simulink model "simulink_qpsk_mrc"  (R2022b)
settings: Solver=VariableStepAuto  StartTime=0.0  StopTime=0  RelTol=1e-3
values from neighbouring files (symbols this model uses):
  n_sd = 1/sqrt(snrlin)    [sim_qpsk_mrc.m]    (also in task2.m = 1./sqrt(snr_lin(i)); task3.m = n(i))
settings Model: Creator=DSP-29  LastModifiedBy=DSP-29

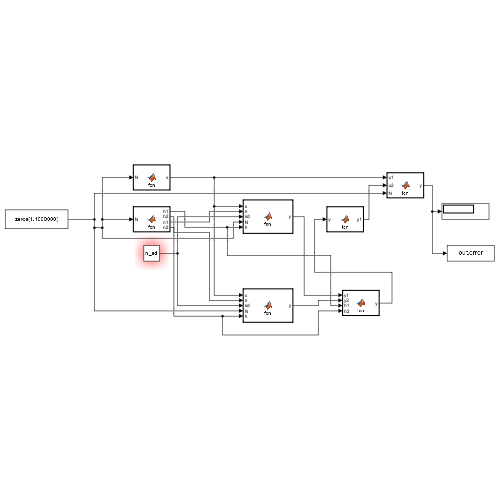
[thumbnail: Simulink's stored preview of the top-level diagram]
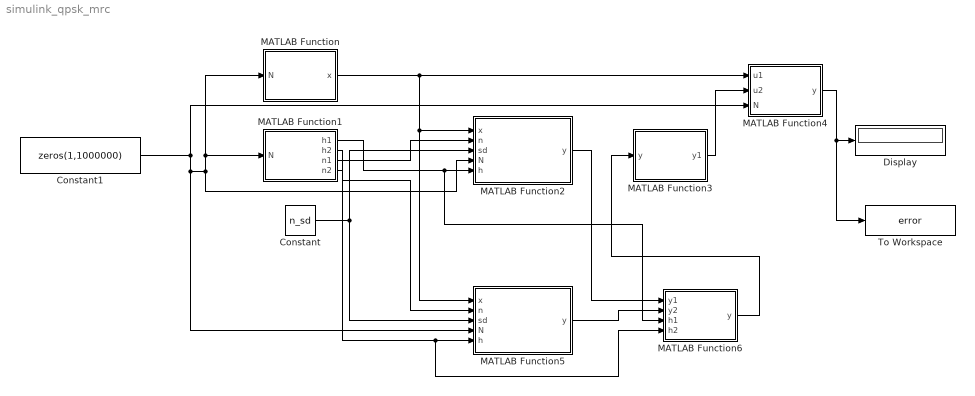
== system simulink_qpsk_mrc ==
  Constant : Constant  Value=n_sd
  Constant1 : Constant  Value=zeros(1,1000000)
  Display : Display
  MATLAB Function : MATLAB Function  TreatAsAtomicUnit=on
  MATLAB Function1 : MATLAB Function  TreatAsAtomicUnit=on
  MATLAB Function2 : MATLAB Function  TreatAsAtomicUnit=on
  MATLAB Function3 : MATLAB Function  TreatAsAtomicUnit=on
  MATLAB Function4 : MATLAB Function  TreatAsAtomicUnit=on
  MATLAB Function5 : MATLAB Function  TreatAsAtomicUnit=on
  MATLAB Function6 : MATLAB Function  TreatAsAtomicUnit=on
  To Workspace : ToWorkspace  VariableName=error  SampleTime=-1
      settings: Save2DSignal=2-D array (concatenate along first dimension)
  wires:
  MATLAB Function2/1(y) -> MATLAB Function6/1(y1)
  MATLAB Function1/1(h1) -> MATLAB Function6/3(h1), MATLAB Function2/5(h)
  MATLAB Function6/1(y) -> MATLAB Function3/1(y)
  Constant1/1 -> MATLAB Function5/4(N), MATLAB Function/1(N), MATLAB Function1/1(N), MATLAB Function2/4(N), MATLAB Function4/3(N)
  MATLAB Function4/1(y) -> To Workspace/1, Display/1
  MATLAB Function/1(x) -> MATLAB Function5/1(x), MATLAB Function2/1(x), MATLAB Function4/1(u1)
  Constant/1 -> MATLAB Function5/3(sd), MATLAB Function2/3(sd)
  MATLAB Function1/3(n1) -> MATLAB Function2/2(n)
  MATLAB Function3/1(y1) -> MATLAB Function4/2(u2)
  MATLAB Function5/1(y) -> MATLAB Function6/2(y2)
  MATLAB Function1/2(h2) -> MATLAB Function6/4(h2), MATLAB Function5/5(h)
  MATLAB Function1/4(n2) -> MATLAB Function5/2(n)

== matlab function simulink_qpsk_mrc/MATLAB Function1 ==
  data: h1 output; h2 output; N input; n1 output; n2 output
function [h1, h2, n1, n2] = fcn(N)
N = length(N);
n1 = complex(randn(1,N),randn(1,N));
h1 = complex(randn(1,N),randn(1,N));
n2 = complex(randn(1,N),randn(1,N));
h2 = complex(randn(1,N),randn(1,N));

== matlab function simulink_qpsk_mrc/MATLAB Function ==
  data: x output; N input
function x  = fcn(N)
N = length(N);
x = randi([0 1], 1 , N) + 1j*randi([0 1], 1, N);
x = 2*x - (1+1j); x = x/sqrt(2);

== matlab function simulink_qpsk_mrc/MATLAB Function2 ==
  data: x input; y output; n input; sd input; N input; h input
function y  = fcn(x,n,sd,N,h)
N = length(N);
y = complex(zeros(1,N),zeros(1,N)); %initialize
y = (h.*x)+(n*sd);

== matlab function simulink_qpsk_mrc/MATLAB Function3 ==
  data: y input; y1 output
function y1 = fcn(y)
y1 = 2*(real(y)>0) - 1 + 1j*(2*(imag(y)>0)-1);
y1 = y1/sqrt(2);

== matlab function simulink_qpsk_mrc/MATLAB Function4 ==
  data: u1 input; y output; u2 input; N input
function y = fcn(u1,u2,N)
N = length(N);
y = (sum(abs(u1-u2)))/N;

== matlab function simulink_qpsk_mrc/MATLAB Function5 ==
  data: x input; y output; n input; sd input; N input; h input
function y  = fcn(x,n,sd,N,h)
N = length(N);
y = complex(zeros(1,N),zeros(1,N)); %initialize
y = (h.*x)+(n*sd);

== matlab function simulink_qpsk_mrc/MATLAB Function6 ==
  data: y1 input; y output; y2 input; h1 input; h2 input
function y = fcn(y1, y2, h1, h2)
mrc_y = conj(h1).*y1 + conj(h2).*y2;
y = mrc_y./(h1.*conj(h1) + h2.*conj(h2));
